simulink model "flags_task"  (Simulink 3.00)
libraries: mathlib x11, inoutlib x4

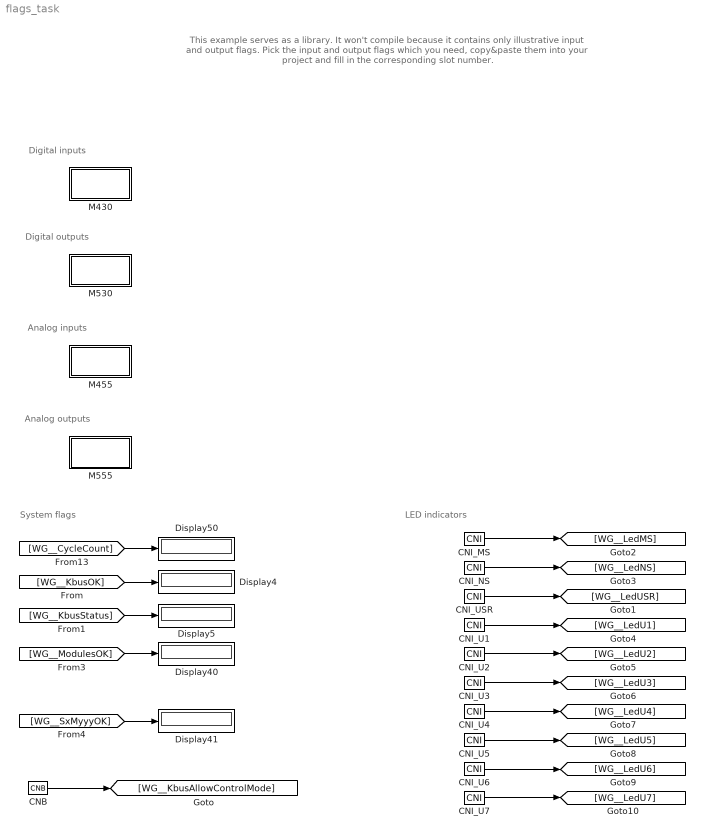
== system flags_task ==
  note: This example serves as a library. It won't compile because it contains only illustrative
      | input and output flags.
      | Pick the input and output flags which you need, copy&paste them into your project
      | and fill in the corresponding slot number.
  note: System flags
  note: LED indicators
  note: Digital inputs
  note: Digital outputs
  note: Analog outputs
  note: Analog inputs
  CNB : mathlib/CNB  YCN=off
  CNI_MS : mathlib/CNI  icn=0
  CNI_NS : mathlib/CNI  icn=0
  CNI_U{1..7} (7 alike) : mathlib/CNI  icn=0
  CNI_USR : mathlib/CNI  icn=0
  Display{4..5,40..41,50} (5 alike) : Display
      settings: Format=Best fit
  M430 : Subsystem
      mask Type: REX sequence
  M455 : Subsystem
      mask Type: REX sequence
  M530 : Subsystem
      mask Type: REX sequence
  M555 : Subsystem
      mask Type: REX sequence
  wires:
  CNB/1 -> [WG__KbusAllowControlMode]
  CNI_MS/1 -> [WG__LedMS]
  CNI_NS/1 -> [WG__LedNS]
  CNI_U1/1 -> [WG__LedU1]
  CNI_U2/1 -> [WG__LedU2]
  CNI_U3/1 -> [WG__LedU3]
  CNI_U4/1 -> [WG__LedU4]
  CNI_U5/1 -> [WG__LedU5]
  CNI_U6/1 -> [WG__LedU6]
  CNI_U7/1 -> [WG__LedU7]
  CNI_USR/1 -> [WG__LedUSR]
  [WG__KbusOK] -> Display4/1
  [WG__KbusStatus] -> Display5/1
  [WG__CycleCount] -> Display50/1
  [WG__ModulesOK] -> Display40/1
  [WG__SxMyyyOK] -> Display41/1

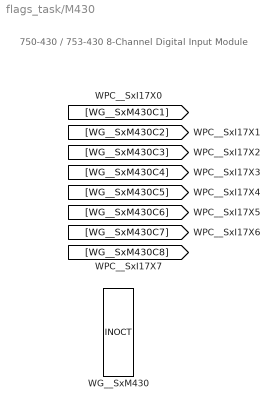
== system flags_task/M430 ==
  note: 750-430 / 753-430
      | 8-Channel Digital Input Module
  WG__SxM430 : inoutlib/INOCT

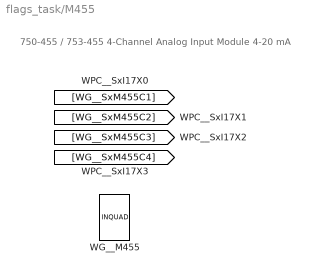
== system flags_task/M455 ==
  note: 750-455 / 753-455
      | 4-Channel Analog Input Module 4-20 mA
  WG__M455 : inoutlib/INQUAD

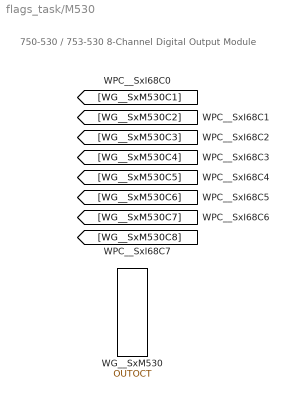
== system flags_task/M530 ==
  note: 750-530 / 753-530
      | 8-Channel Digital Output Module
  WG__SxM530 : inoutlib/OUTOCT

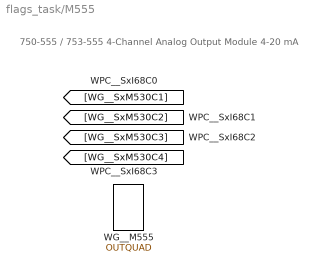
== system flags_task/M555 ==
  note: 750-555 / 753-555
      | 4-Channel Analog Output Module 4-20 mA
  WG__M555 : inoutlib/OUTQUAD
